simulink model "like_a_star_trajectory"  (R2020a)
settings: Solver=VariableStepAuto  StartTime=0.0  StopTime=7  FixedStep=0.0000001  RelTol=1e-3
values from neighbouring files (symbols this model uses):
  L = 1.760    (= 1.76)    [Parameters.m]
  Vz = 0    [Parameters.m]
libraries: simulink x6
settings Model: PauseTimes=3  Creator=Eugene  LastModifiedBy=corsair
settings DataIOCC: ReturnWorkspaceOutputs=off
settings DebuggingCC: ParameterOverflowMsg=warning  ArithmeticOperatorsInVariantConditions=warning
settings HardwareCC: ProdHWDeviceType=AMD->x86-64 (Windows64)
settings SFSimCC: SimUseLocalCustomCode=off  CustomCodeUndefinedFunction=UseInterfaceOnly
settings RTWCC: RTWUseLocalCustomCode=off

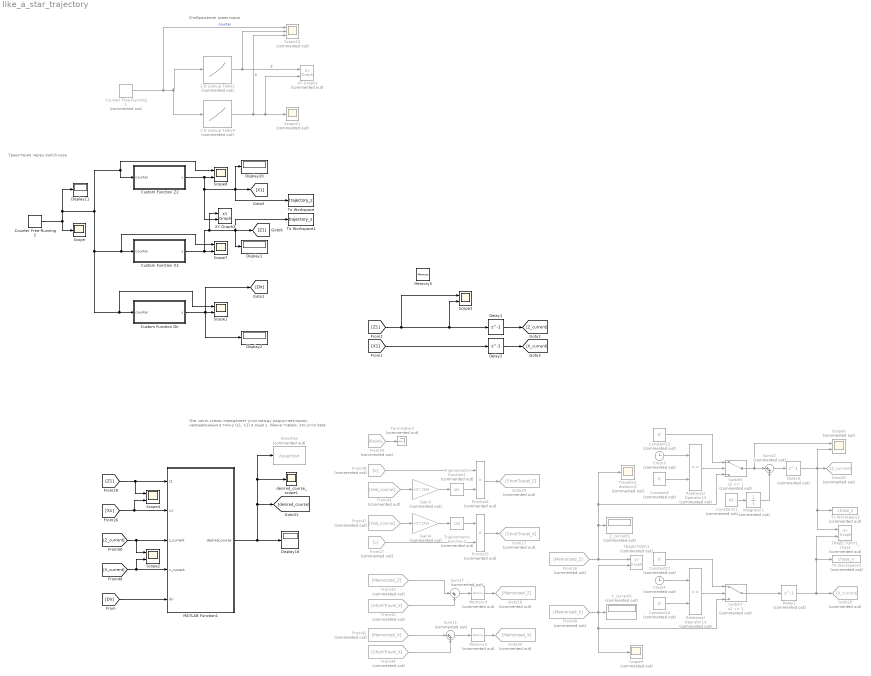
== system like_a_star_trajectory ==
  note: Траектория через switch-case
  note: Отображение траектории
  note: Эта часть схемы определяет угол между радиус-вектором, направленным в точку (z1, x1) и осью z. Иначе говоря, это угол beta
  1-D Lookup Table1 : Lookup_n-D  Commented=on  NumberOfTableDimensions=1  BreakpointsForDimension1=[0:7]  BreakpointsForDimension1FirstPoint=0  BreakpointsForDimension1DataTypeStr=uint8  Table=[0,0,L,L,2*L,2*L,3*L, 3*L]  TableDataTypeStr=double  InterpMethod=Flat  ExtrapMethod=Cubic spline  RemoveProtectionInput=on  InternalRulePriority=Speed  OutDataTypeStr=double  RndMeth=Zero  InputSameDT=on
  1-D Lookup Table4 : Lookup_n-D  Commented=on  NumberOfTableDimensions=1  BreakpointsForDimension1=[0:7]  BreakpointsForDimension1DataTypeStr=int16  Table=[0,25,25,0,0,25,25,0]  TableDataTypeStr=double  InterpMethod=Flat  RemoveProtectionInput=on  InternalRulePriority=Speed  OutDataTypeStr=double  RndMeth=Zero  InputSameDT=on
  Assertion : Assertion  Commented=on  AssertionFailFcn=-1
  Clock3 : Clock  Commented=on
  Clock4 : Clock  Commented=on
  Constant11 : Constant  Commented=on  Value=Vz
  Constant{2,15..17} (4 alike) : Constant  Commented=on  Value=0
  Counter Free-Running1 : simulink/Sources/Counter Free-Running  Commented=on  NumBits=3  tsamp=1
  Counter Free-Running2 : simulink/Sources/Counter Free-Running  NumBits=3  tsamp=1
  Custom Function Dir : MATLAB Function  TreatAsAtomicUnit=on
  Custom Function X2 : MATLAB Function  TreatAsAtomicUnit=on
  Custom Function Z2 : MATLAB Function  TreatAsAtomicUnit=on
  Delay1 : Delay  DelayLength=1  SampleTime=1
  Delay2 : Delay  DelayLength=1  InitialCondition=13  SampleTime=1
  Delay5 : Delay  Commented=on  DelayLength=1  SampleTime=0.05
  Delay6 : Delay  Commented=on  DelayLength=1  SampleTime=0.05
  Display{1..2,11,16,20} (5 alike) : Display
  From16 : From  Commented=on  GotoTag=Memorized_Z
  From27 : From  Commented=on  GotoTag=L
  From28 : From  Commented=on  GotoTag=L
  From32 : From  Commented=on  GotoTag=ShortTravel_Z
  From33 : From  Commented=on  GotoTag=Memorized_Z
  From34 : From  Commented=on  GotoTag=Reset
  From43 : From  Commented=on  GotoTag=real_course
  From44 : From  Commented=on  GotoTag=ShortTravel_X
  From45 : From  Commented=on  GotoTag=Memorized_X
  From47 : From  Commented=on  GotoTag=real_course
  From48 : From  Commented=on  GotoTag=Memorized_X
  Gain3 : Gain  Commented=on  Gain=1/57.2958
  Gain4 : Gain  Commented=on  Gain=1/57.2958
  Goto16 : Goto  Commented=on  GotoTag=Memorized_Z
  Goto17 : Goto  Commented=on  GotoTag=ShortTravel_X
  Goto20 : Goto  Commented=on  GotoTag=ShortTravel_Z
  Goto28 : Goto  Commented=on  GotoTag=Z_current
  Goto29 : Goto  Commented=on  GotoTag=X_current
  Goto30 : Goto  Commented=on  GotoTag=Memorized_X
  Integrator1 : Integrator  Commented=on
  MATLAB Function1 : MATLAB Function  TreatAsAtomicUnit=on
  Memory3 : Memory  Commented=on  InitialCondition=15
  Memory4 : Memory  Commented=on
  Memory5 : Memory
  Product4 : Product  Commented=on
  Product5 : Product  Commented=on
  Relational Operator13 : RelationalOperator  Commented=on  Operator===  OutDataTypeStr=boolean  RndMeth=Simplest
  Relational Operator14 : RelationalOperator  Commented=on  Operator===  OutDataTypeStr=boolean  RndMeth=Simplest
  Scope : Scope
  Scope{1..4,7..8} (6 alike) : Scope  NumInputPorts=2
  Scope10 : Scope  Commented=on  NumInputPorts=3
  Scope11 : Scope  Commented=on
  Scope6 : Scope  Commented=on  NumInputPorts=2
  Scope9 : Scope  Commented=on
  Sum10 : Sum  Commented=on  Inputs=|++
  Sum11 : Sum  Commented=on  Inputs=|++
  Sum17 : Sum  Commented=on  Inputs=|++
  Switch6 : Switch  Commented=on  Threshold=1
  Switch7 : Switch  Commented=on  Threshold=1
  TRAJECTORY1 : simulink/Sinks/XY Graph  Commented=on  xmin=-1  xmax=10  ymin=-5  ymax=30  st=-1
  TRAJECTORY1_chase : simulink/Sinks/XY Graph  Commented=on  xmin=-15  xmax=15  ymin=-15  ymax=15  st=-1
  Terminator3 : Terminator  Commented=on
  To Workspace : ToWorkspace  VariableName=trajectory_z  SampleTime=-1
  To Workspace1 : ToWorkspace  VariableName=trajectory_x  SampleTime=-1
  To Workspace2 : ToWorkspace  Commented=on  VariableName=chase_z  SampleTime=-1
  To Workspace3 : ToWorkspace  Commented=on  VariableName=chase_x  SampleTime=-1
  Travelled_distance1 : Scope  Commented=on
  Trigonometric Function2 : Trigonometry  Commented=on
  Trigonometric Function3 : Trigonometry  Commented=on  Operator=cos
  XY Graph2 : simulink/Sinks/XY Graph  Commented=on  xmin=-10  xmax=20  ymin=-10  ymax=30  st=-1
  XY Graph3 : simulink/Sinks/XY Graph  xmin=-15  xmax=15  ymin=-15  ymax=15  st=-1
  X_current1 : Display  Commented=on
  Z_current1 : Display  Commented=on
  desired_course_scope1 : Scope
  wires:
  Counter Free-Running2/1 -> Display11/1, Scope1/1, Custom Function Dir/1(counter), Scope7/1, Custom Function X2/1(counter), Scope8/1, Custom Function Z2/1(counter), Scope/1
  1-D Lookup Table1/1 -> XY Graph2/1, Scope10/2  "Z"
  1-D Lookup Table4/1 -> Scope11/1, XY Graph2/2, Scope10/3  "X"
  Counter Free-Running1/1 -> Scope10/1, 1-D Lookup Table1/1, 1-D Lookup Table4/1  "counter"
  Custom Function Z2/1(y) -> Scope8/2, XY Graph3/2, [X1], To Workspace/1, Display20/1
  Custom Function X2/1(y) -> XY Graph3/1, [Z1], To Workspace1/1, Display1/1, Scope7/2
  Custom Function Dir/1(y) -> Display2/1, [Dir], Scope1/2
  [Z1] -> Scope4/1, MATLAB Function1/1(z1)
  [X_current] -> Scope2/2, MATLAB Function1/4(x_current)
  [X1] -> MATLAB Function1/2(x1), Scope4/2
  [Z_current] -> MATLAB Function1/3(z_current), Scope2/1
  MATLAB Function1/1(desired_course) -> [desired_course], Assertion/1, desired_course_scope1/1, Display16/1
  Sum17/1 -> Memory4/1
  Trigonometric Function2/1 -> Product4/2
  Switch6/1 -> Scope6/1, Sum10/1
  Memory3/1 -> Goto30/1
  From43/1 -> Gain3/1
  Product4/1 -> Goto20/1
  Sum11/1 -> Memory3/1
  From33/1 -> Sum17/1
  Gain3/1 -> Trigonometric Function2/1
  Constant11/1 -> Integrator1/1
  From47/1 -> Gain4/1
  Constant17/1 -> Switch7/1
  Memory4/1 -> Goto16/1
  From16/1 -> Switch6/3, Travelled_distance1/1, Z_current1/1, TRAJECTORY1/1
  Clock4/1 -> Relational Operator14/1
  From44/1 -> Sum11/2
  From34/1 -> Terminator3/1
  Trigonometric Function3/1 -> Product5/1
  Clock3/1 -> Relational Operator13/1
  Delay6/1 -> TRAJECTORY1_chase/1, To Workspace2/1, Goto28/1, Scope6/2
  Sum10/1 -> Delay6/1
  Relational Operator13/1 -> Switch6/2
  Constant16/1 -> Relational Operator14/2
  Gain4/1 -> Trigonometric Function3/1
  From32/1 -> Sum17/2
  Delay5/1 -> Goto29/1, TRAJECTORY1_chase/2, To Workspace3/1
  Integrator1/1 -> Sum10/2
  From27/1 -> Product5/2
  Product5/1 -> Goto17/1
  From28/1 -> Product4/1
  From45/1 -> Sum11/1
  Constant2/1 -> Relational Operator13/2
  Switch7/1 -> Delay5/1
  From48/1 -> Switch7/3, Scope9/1, TRAJECTORY1/2, X_current1/1
  Constant15/1 -> Switch6/1
  Relational Operator14/1 -> Switch7/2
  [X1] -> Delay2/1
  [Z1] -> Scope3/2, Delay1/1, Scope3/1
  Delay1/1 -> [Z_current]
  Delay2/1 -> [X_current]
  [Dir] -> MATLAB Function1/5(dir)

== matlab function like_a_star_trajectory/Custom Function X2 ==
  data: counter input; y output
function y = fcn(counter)

%L = 1.76;

switch counter
   
    case 1
      y = -0.76;
    case 2
        y = -3.36;
    case 3
      y = -2.22;
    case 4
      y = -6.5;
    case 5
      y = -3.53;
    case 6
      y = -9.19;
    case 7
        y = -4.6;
   otherwise
      y = 0;

end

== matlab function like_a_star_trajectory/Custom Function Z2 ==
  data: counter input; y output
function y = fcn( counter)

%L = 1.76;



switch counter
    case 1
      y = 5.75;
    case 2
      y = 12.56;
    case 3
      y = 5.36;
    case 4
      y = 11.26;
    case 5
      y = 4.6;
    case 6
      y = 9.19;
    case 7
      y = 3.53;
     
   otherwise
      y = 13;
end

== matlab function like_a_star_trajectory/Custom Function Dir ==
  data: counter input; y output
function y = fcn(counter)

%L = 1.76;
% 1 - fwd, -1 - backward

    if mod(int32(counter), 2) == 1
        y = 1;
    else
        y = -1;
    end
end

== matlab function like_a_star_trajectory/MATLAB Function1 ==
  data: z1 input; x1 input; z_current input; desired_course output; x_current input; dir input
function desired_course = fcn(z1, x1, z_current, x_current, dir)

delta_x = x1 - x_current;
delta_z = z1 - z_current;

%1
if (delta_x >= 0) && (delta_z >= 0)
    desired_course = 57.2958*atan(delta_z / delta_x);
%2    
elseif (delta_x >= 0) && (delta_z < 0)
    desired_course = 360 - 57.2958*atan( abs(delta_z) / delta_x);
%3    
elseif (delta_x < 0) && (delta_z < 0)    
    desired_course = 180 + 57.2958*atan(abs(delta_z) / abs(delta_x));
%4    
elseif (delta_x < 0) && (delta_z >= 0)    
    desired_course = 180 - 57.2958*atan( delta_z / abs(delta_x));   
    
else 
    desired_course = -1;
end

    
% При движении назад отнимаем от 360-и    
if dir == -1
    desired_course = desired_course - 180;
end
    
end
